simulink model "emr4_eaxle"  (R2026a)
settings: Solver=VariableStepAuto  StopTime=t_stop
values from neighbouring files (symbols this model uses):
  eta_em_inv = 0.94    [emr4_eaxle_params.m]
  eta_red = 0.97    [emr4_eaxle_params.m]
  i_gear = 11.64    [emr4_eaxle_params.m]
  I_inv_rated = 550    [emr4_eaxle_params.m]
  m_veh = 2300    [emr4_eaxle_params.m]
  P_peak = 155e3    (= 155000)    [emr4_eaxle_params.m]
  r_wheel = 0.35    [emr4_eaxle_params.m]
  radps2rpm = 60/(2*pi)    (= 9.54929658551)    [emr4_eaxle_params.m]
  T_motor_max = 255    [emr4_eaxle_params.m]
  V_dc_nom = 400    [emr4_eaxle_params.m]
  v_init = 0    [emr4_eaxle_params.m]
  v_sat_upper = 1.05 * v_top    (= 52.899670112)    [emr4_eaxle_params.m]
  w_eps = 1    [emr4_eaxle_params.m]
  w_motor_max = n_motor_max * 2*pi/60    (= 1675.51608191)    [emr4_eaxle_params.m]
libraries: hdlsllib x2
settings Model: Creator=Razvan  LastModifiedBy=Razvan

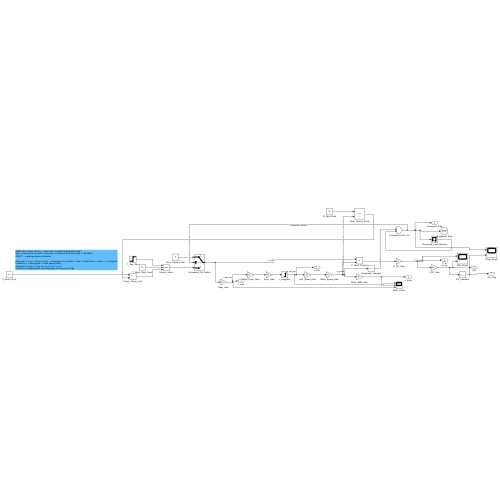
[thumbnail: Simulink's stored preview of the top-level diagram]
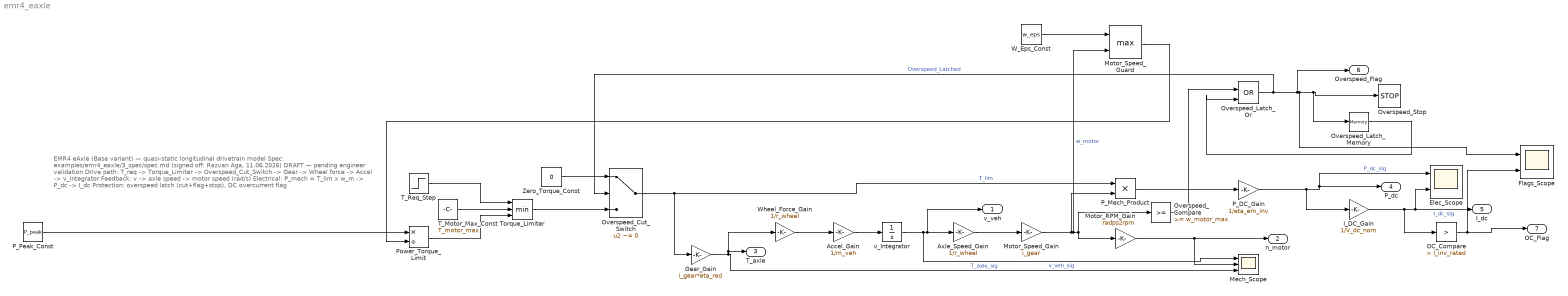
== system emr4_eaxle ==
  note: EMR4 eAxle (Base variant) — quasi-static longitudinal drivetrain model
      | Spec: examples/emr4_eaxle/3_spec/spec.md (signed off: Razvan Aga, 11.06.2026)
      | DRAFT — pending engineer validation
      |
      | Drive path: T_req -> Torque_Limiter -> Overspeed_Cut_Switch -> Gear -> Wheel force -> Accel -> v_Integrator
      | Feedback: v -> axle speed -> motor speed (rad/s)
      | Electrical: P_mech = T_lim x w_m -> P_dc -> I_dc
      | Protection: overspeed latch (cut+flag+stop), DC overcurrent flag
  Accel_Gain : Gain  Description=Spec §3 m_veh = 2300 kg (ASSUMED, §9.4); a = F / m (§4)  Gain=1/m_veh
  Axle_Speed_Gain : Gain  Description=Spec §3 r_wheel; w_axle = v / r_wheel (config feedback path)  Gain=1/r_wheel
  Elec_Scope : Scope  NumInputPorts=2
      settings: Description=P_dc, I_dc
  Flags_Scope : Scope  NumInputPorts=2
      settings: Description=Overspeed_Flag, OC_Flag
  Gear_Gain : Gain  Description=Spec §3 i_gear = 11.64 (ASSUMED, §9.2) x eta_red = 0.97 (ASSUMED, §9.3); config drive path  Gain=i_gear*eta_red
  I_DC_Gain : Gain  Description=Spec §3 V_dc_nom = 400 V (ASSUMED); I_dc = P_dc / V_dc_nom (§4)  Gain=1/V_dc_nom
  Mech_Scope : Scope  NumInputPorts=3
      settings: Description=v_veh, n_motor, T_axle
  Motor_RPM_Gain : Gain  Description=Unit conversion rad/s -> rpm (params file radps2rpm)  Gain=radps2rpm
  Motor_Speed_Gain : Gain  Description=Spec §3 i_gear; w_m = w_axle x i (config feedback path)  Gain=i_gear
  Motor_Speed_Guard : MinMax  Description=Implementation guard: w_safe = max(w_m, w_eps) for P/w division  Function=max  Inputs=2
  OC_Compare : hdlsllib/Logic and Bit Operations/Compare To Constant  Description=Spec §5: DC overcurrent check I_dc > 550 A (I_inv_rated, VMS p.8) -> flag; should never assert (AC6)  relop=>  const=I_inv_rated  OutDataTypeStr=boolean
  Overspeed_Compare : hdlsllib/Logic and Bit Operations/Compare To Constant  Description=Spec §5: motor overspeed w_m >= 16000 rpm (w_motor_max, VMS p.9-10)  relop=>=  const=w_motor_max  OutDataTypeStr=boolean
  Overspeed_Cut_Switch : Switch  Description=Spec §5: overspeed latched -> torque cut to 0 (latched)  Criteria=u2 ~= 0
  Overspeed_Latch_Memory : Memory  Description=Latch state memory, initial 0 (not tripped)
  Overspeed_Latch_Or : Logic  Description=Spec §5: overspeed latch (OR with Memory feedback) — cut is latched  Operator=OR  IconShape=distinctive  AllPortsSameDT=off  OutDataTypeStr=boolean
  Overspeed_Stop : Stop  Description=Spec §6 stop condition: overspeed cut stops simulation
  P_DC_Gain : Gain  Description=Spec §3 eta_em_inv = 0.94 (ASSUMED, §9.3); P_dc = P_mech / eta  Gain=1/eta_em_inv
  P_Mech_Product : Product  Description=Config electrical path: P_mech = T_lim x w_m
  P_Peak_Const : Constant  Description=Spec §3 P_peak = 155 kW (VMS p.7 Fig.2; open item §9.1)  Value=P_peak
  Power_Torque_Limit : Product  Description=Spec §5 power limiting: T = P_peak / w_m (saturation via P/w characteristic)  Inputs=*/
  T_Motor_Max_Const : Constant  Description=Spec §3 T_motor_max = 255 Nm (VMS p.9 reducer input limit)  Value=T_motor_max
  T_Req_Step : Step  Description=Spec §6: torque request step 300 Nm at t=0 (T_req_step), deliberately > T_motor_max to exercise limiter  Time=0  FinalValue=T_req_step  SampleTime=0
  Torque_Limiter : MinMax  Description=Spec §5 + config: T_lim = min(T_req, T_motor_max, P_peak/w_m)  Inputs=3
  W_Eps_Const : Constant  Description=Implementation guard (params file): divide-by-zero protection for P/w branch at standstill; NOT a spec value  Value=w_eps
  Wheel_Force_Gain : Gain  Description=Spec §3 r_wheel = 0.35 m (ASSUMED, §9.4); F = T_axle / r_wheel (§4)  Gain=1/r_wheel
  Zero_Torque_Const : Constant  Description=Spec §5: overspeed latched -> torque cut to 0  Value=0
  v_Integrator : Integrator  Description=Spec §6 IC v=0; saturation guard 0..1.05x top speed (§4) per skill hard rule 4 — overspeed cut acts first  InitialCondition=v_init  LimitOutput=on  UpperSaturationLimit=v_sat_upper  LowerSaturationLimit=0
  v_veh : Outport  Description=Spec §6 output: vehicle speed m/s
  n_motor : Outport  Description=Spec §6 output: motor speed rpm  Port=2
  T_axle : Outport  Description=Spec §6 output: axle torque Nm  Port=3
  P_dc : Outport  Description=Spec §6 output: DC-link power W  Port=4
  I_dc : Outport  Description=Spec §6 output: DC-link current A  Port=5
  Overspeed_Flag : Outport  Description=Spec §5/§6 output: overspeed latch flag  Port=6
  OC_Flag : Outport  Description=Spec §5/§6 output: DC overcurrent flag  Port=7
  wires:
  T_Req_Step/1 -> Torque_Limiter/1
  T_Motor_Max_Const/1 -> Torque_Limiter/2
  P_Peak_Const/1 -> Power_Torque_Limit/1
  W_Eps_Const/1 -> Motor_Speed_Guard/1
  Motor_Speed_Gain/1 -> Overspeed_Compare/1, Motor_RPM_Gain/1, Motor_Speed_Guard/2, P_Mech_Product/2  "w_motor"
  Motor_Speed_Guard/1 -> Power_Torque_Limit/2
  Power_Torque_Limit/1 -> Torque_Limiter/3
  Zero_Torque_Const/1 -> Overspeed_Cut_Switch/1
  Overspeed_Latch_Or/1 -> Overspeed_Stop/1, Overspeed_Latch_Memory/1, Flags_Scope/1, Overspeed_Flag/1, Overspeed_Cut_Switch/2  "Overspeed_Latched"
  Torque_Limiter/1 -> Overspeed_Cut_Switch/3
  Overspeed_Cut_Switch/1 -> P_Mech_Product/1, Gear_Gain/1  "T_lim"
  Gear_Gain/1 -> Wheel_Force_Gain/1, T_axle/1, Mech_Scope/3  "T_axle_sig"
  Wheel_Force_Gain/1 -> Accel_Gain/1
  Accel_Gain/1 -> v_Integrator/1
  v_Integrator/1 -> v_veh/1, Axle_Speed_Gain/1, Mech_Scope/1  "v_veh_sig"
  Axle_Speed_Gain/1 -> Motor_Speed_Gain/1
  P_Mech_Product/1 -> P_DC_Gain/1
  P_DC_Gain/1 -> P_dc/1, Elec_Scope/1, I_DC_Gain/1  "P_dc_sig"
  Overspeed_Compare/1 -> Overspeed_Latch_Or/1
  Overspeed_Latch_Memory/1 -> Overspeed_Latch_Or/2
  I_DC_Gain/1 -> Elec_Scope/2, I_dc/1, OC_Compare/1  "I_dc_sig"
  Motor_RPM_Gain/1 -> Mech_Scope/2, n_motor/1
  OC_Compare/1 -> Flags_Scope/2, OC_Flag/1
